simulink model "wheelleg_simulator"  (R2024b)
settings: Solver=VariableStepAuto  StartTime=0.0  StopTime=15.0  RelTol=1e-3
undefined symbols (not defined in the file): eta_l, g, mb, ml, Rl, X, Y, Z
libraries: sm_lib x92, nesl_utility x27, simulink x8, slpidlib x2
(part 1 of 3)
settings Model: Creator=Ame  LastModifiedBy=Ame

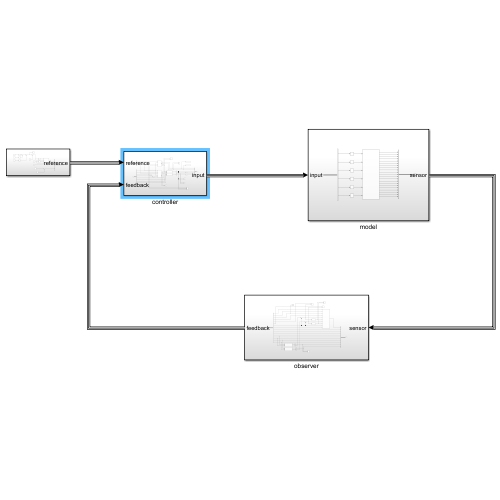
[thumbnail: Simulink's stored preview of the top-level diagram]
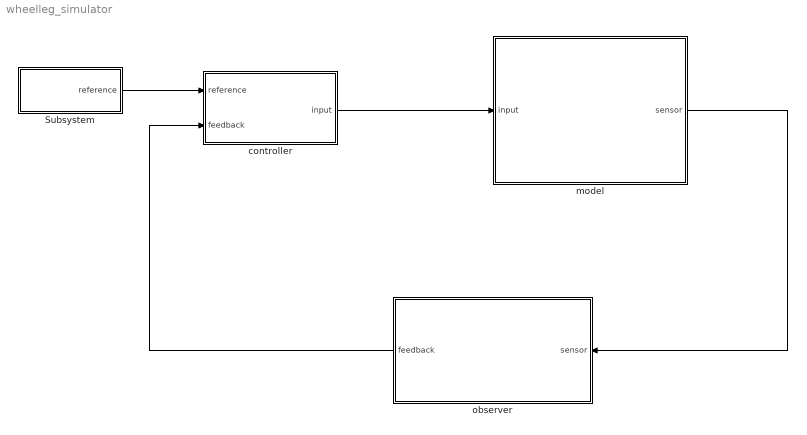
== system wheelleg_simulator ==
  Subsystem : Subsystem
  controller : Subsystem
  model : Subsystem
  observer : Subsystem
  wires:
  model/1(sensor) -> observer/1(sensor)
  observer/1(feedback) -> controller/2(feedback)
  controller/1(input) -> model/1(input)
  Subsystem/1(reference) -> controller/1(reference)

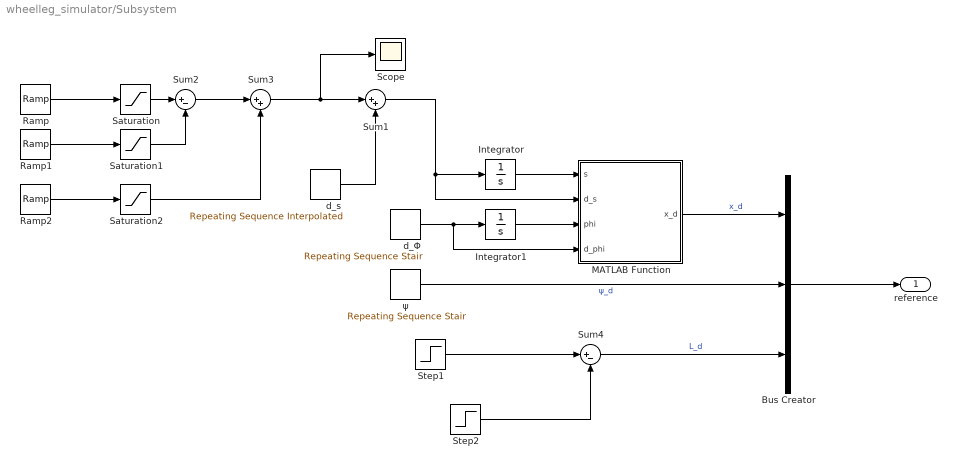
== system wheelleg_simulator/Subsystem ==
  Bus Creator : BusCreator  Inputs=3
  Integrator : Integrator
  Integrator1 : Integrator
  MATLAB Function : MATLAB Function  TreatAsAtomicUnit=on
  Ramp : simulink/Sources/Ramp  slope=0.3  start=0  InitialOutput=0
  Ramp1 : simulink/Sources/Ramp  slope=0.3  start=12  InitialOutput=0
  Ramp2 : simulink/Sources/Ramp  slope=0.3  start=5.5  InitialOutput=0
  Saturation : Saturate  UpperLimit=1.5
  Saturation1 : Saturate  UpperLimit=1  LowerLimit=-0.21
  Saturation2 : Saturate  UpperLimit=0.6
  Scope : Scope
  Step1 : Step  Time=9.0  Before=0.25  After=0.45  SampleTime=0
  Step2 : Step  Time=9.15  After=0.2  SampleTime=0
  Sum1 : Sum  Inputs=|++
  Sum2 : Sum  Inputs=|+-
  Sum3 : Sum  Inputs=|++
  Sum4 : Sum  Inputs=|+-
  d_s : simulink/Sources/Repeating Sequence Interpolated  OutValues=[0 0 0 0 0 0].'  TimeValues=[0 2 3 4 5 6 ].'  LookUpMeth=Interpolation-Use End Values  tsamp=0.01  OutMin=[]  OutMax=[]  OutDataTypeStr=double  OutputDataTypeScalingMode=double  OutDataType=fixdt(0,8)  OutScaling=2^-10
  d_Φ : simulink/Sources/Repeating Sequence Stair  OutValues=[0].'  tsamp=2  OutMin=[]  OutMax=[]  OutDataTypeStr=double  OutputDataTypeScalingMode=double  OutDataType=fixdt(0,8)  ConRadixGroup=Best Precision: Vector-wise  OutScaling=2^-12
  ψ : simulink/Sources/Repeating Sequence Stair  OutValues=[0].'  tsamp=2  OutMin=[]  OutMax=[]  OutDataTypeStr=double  OutputDataTypeScalingMode=double  OutDataType=fixdt(0,8)  ConRadixGroup=Best Precision: Vector-wise  OutScaling=2^-12
  reference : Outport
  wires:
  Bus Creator/1 -> reference/1
  MATLAB Function/1(x_d) -> Bus Creator/1  "x_d"
  ψ/1 -> Bus Creator/2  "ψ_d"
  Integrator/1 -> MATLAB Function/1(s)
  d_Φ/1 -> MATLAB Function/4(d_phi), Integrator1/1
  Integrator1/1 -> MATLAB Function/3(phi)
  Ramp/1 -> Saturation/1
  d_s/1 -> Sum1/2
  Sum1/1 -> MATLAB Function/2(d_s), Integrator/1
  Saturation/1 -> Sum2/1
  Ramp1/1 -> Saturation1/1
  Saturation1/1 -> Sum2/2
  Step1/1 -> Sum4/1
  Sum4/1 -> Bus Creator/3  "L_d"
  Step2/1 -> Sum4/2
  Saturation2/1 -> Sum3/2
  Ramp2/1 -> Saturation2/1
  Sum2/1 -> Sum3/1
  Sum3/1 -> Scope/1, Sum1/1

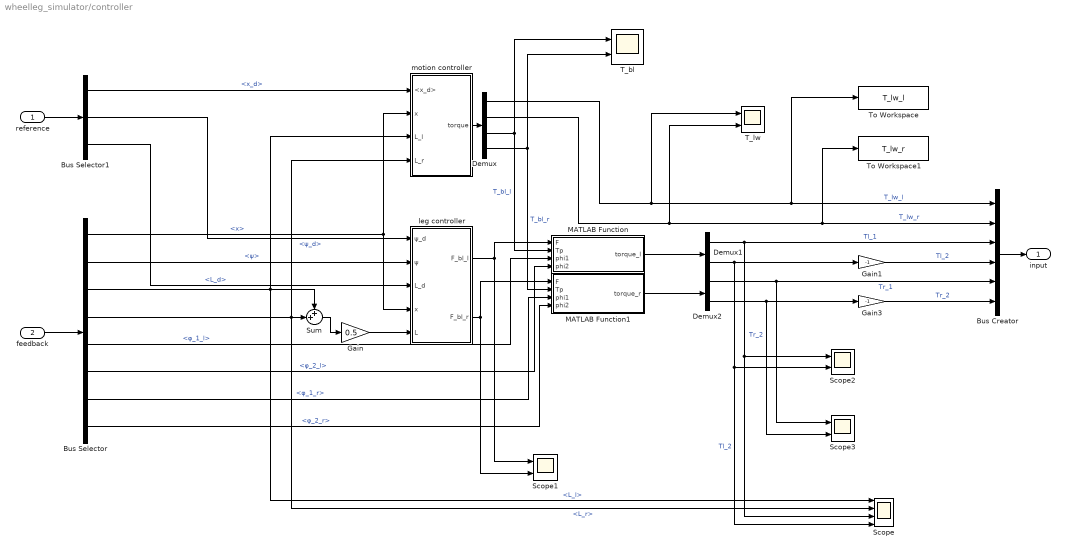
== system wheelleg_simulator/controller ==
  reference : Inport
  feedback : Inport  Port=2
  Bus Creator : BusCreator  Inputs=6
  Bus Selector : BusSelector  OutputSignals=x,ψ,L_l,L_r,φ_1_l,φ_2_l,φ_1_r,φ_2_r
  Bus Selector1 : BusSelector  OutputSignals=x_d,ψ_d,L_d
  Demux : Demux
  Demux1 : Demux  Outputs=2
  Demux2 : Demux  Outputs=2
  Gain : Gain  Gain=0.5
  Gain1 : Gain  Gain=-1
  Gain3 : Gain  Gain=-1
  MATLAB Function : MATLAB Function  TreatAsAtomicUnit=on
  MATLAB Function1 : MATLAB Function  TreatAsAtomicUnit=on
  Scope : Scope  NumInputPorts=4
  Scope1 : Scope  NumInputPorts=2
  Scope2 : Scope  NumInputPorts=2
  Scope3 : Scope  NumInputPorts=2
  Sum : Sum  Inputs=++|
  T_bl : Scope  NumInputPorts=2
  T_lw : Scope  NumInputPorts=2
  To Workspace : ToWorkspace  VariableName=T_lw_l  SaveFormat=Timeseries  SampleTime=-1
  To Workspace1 : ToWorkspace  VariableName=T_lw_r  SaveFormat=Timeseries  SampleTime=-1
  leg controller : Subsystem
  motion controller : Subsystem
  input : Outport
  wires:
  feedback/1 -> Bus Selector/1
  Bus Selector/1 -> motion controller/2(x), leg controller/4(x)  "<x>"
  Bus Selector/2 -> leg controller/2(ψ)  "<ψ>"
  Bus Selector/3 -> Scope/1, motion controller/3(L_l), Sum/1  "<L_l>"
  Bus Selector/4 -> motion controller/4(L_r), Sum/2, Scope/2  "<L_r>"
  reference/1 -> Bus Selector1/1
  Bus Selector1/1 -> motion controller/1(<x_d>)  "<x_d>"
  Bus Selector1/2 -> leg controller/1(ψ_d)  "<ψ_d>"
  Bus Selector1/3 -> leg controller/3(L_d)  "<L_d>"
  motion controller/1(torque) -> Demux/1
  Demux/1 -> To Workspace/1, Bus Creator/1, T_lw/1  "T_lw_l"
  Demux/3 -> MATLAB Function/2(Tp), T_bl/1  "T_bl_l"
  Demux/4 -> MATLAB Function1/2(Tp), T_bl/2  "T_bl_r"
  Bus Selector/5 -> MATLAB Function/3(phi1)  "<φ_1_l>"
  Bus Selector/6 -> MATLAB Function/4(phi2)  "<φ_2_l>"
  Bus Selector/7 -> MATLAB Function1/3(phi1)  "<φ_1_r>"
  Bus Selector/8 -> MATLAB Function1/4(phi2)  "<φ_2_r>"
  Bus Creator/1 -> input/1
  MATLAB Function/1(torque_l) -> Demux1/1
  MATLAB Function1/1(torque_r) -> Demux2/1
  Demux2/2 -> Scope3/2, Gain3/1  "Tr_2"
  Demux1/1 -> Bus Creator/3, Scope2/1, Scope/3  "Tl_1"
  Demux1/2 -> Scope2/2, Scope/4, Gain1/1  "Tl_2"
  Demux2/1 -> Bus Creator/5, Scope3/1  "Tr_1"
  leg controller/1(F_bl_l) -> MATLAB Function/1(F), Scope1/1
  Demux/2 -> To Workspace1/1, Bus Creator/2, T_lw/2  "T_lw_r"
  leg controller/2(F_bl_r) -> MATLAB Function1/1(F), Scope1/2
  Sum/1 -> Gain/1
  Gain1/1 -> Bus Creator/4  "Tl_2"
  Gain3/1 -> Bus Creator/6  "Tr_2"
  Gain/1 -> leg controller/5(L)

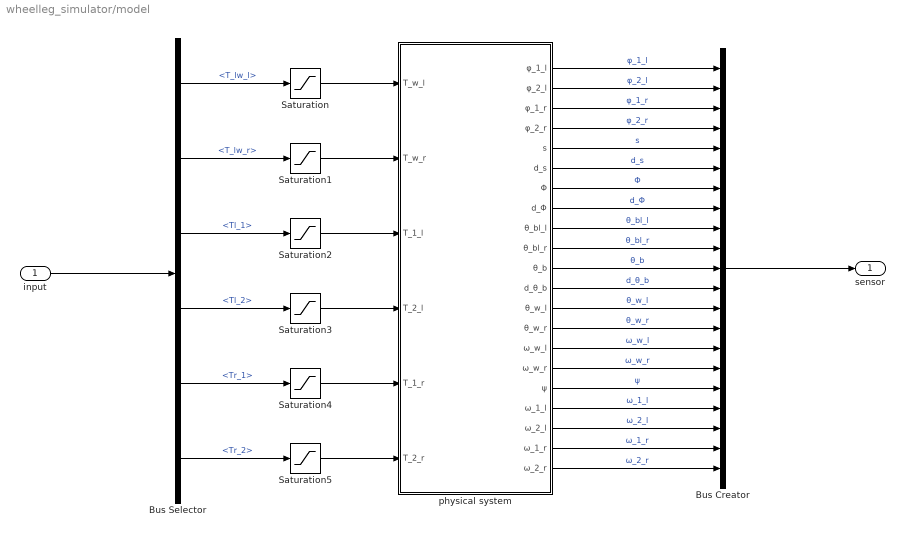
== system wheelleg_simulator/model ==
  input : Inport
  Bus Creator : BusCreator  Inputs=21
  Bus Selector : BusSelector  OutputSignals=T_lw_l,T_lw_r,Tl_1,Tl_2,Tr_1,Tr_2
  Saturation{,1..5} (6 alike) : Saturate  UpperLimit=100  LowerLimit=-100
  physical system : Subsystem
  sensor : Outport
  wires:
  Bus Creator/1 -> sensor/1
  input/1 -> Bus Selector/1
  Bus Selector/1 -> Saturation/1  "<T_lw_l>"
  Bus Selector/2 -> Saturation1/1  "<T_lw_r>"
  physical system/1(φ_1_l) -> Bus Creator/1  "φ_1_l"
  physical system/2(φ_2_l) -> Bus Creator/2  "φ_2_l"
  physical system/3(φ_1_r) -> Bus Creator/3  "φ_1_r"
  physical system/4(φ_2_r) -> Bus Creator/4  "φ_2_r"
  physical system/5(s) -> Bus Creator/5  "s"
  physical system/6(d_s) -> Bus Creator/6  "d_s"
  physical system/7(Φ) -> Bus Creator/7  "Φ"
  physical system/8(d_Φ) -> Bus Creator/8  "d_Φ"
  physical system/9(θ_bl_l) -> Bus Creator/9  "θ_bl_l"
  physical system/10(θ_bl_r) -> Bus Creator/10  "θ_bl_r"
  physical system/11(θ_b) -> Bus Creator/11  "θ_b"
  physical system/12(d_θ_b) -> Bus Creator/12  "d_θ_b"
  physical system/13(θ_w_l) -> Bus Creator/13  "θ_w_l"
  physical system/14(θ_w_r) -> Bus Creator/14  "θ_w_r"
  physical system/15(ω_w_l) -> Bus Creator/15  "ω_w_l"
  physical system/16(ω_w_r) -> Bus Creator/16  "ω_w_r"
  physical system/17(ψ) -> Bus Creator/17  "ψ"
  physical system/18(ω_1_l) -> Bus Creator/18  "ω_1_l"
  physical system/19(ω_2_l) -> Bus Creator/19  "ω_2_l"
  physical system/20(ω_1_r) -> Bus Creator/20  "ω_1_r"
  physical system/21(ω_2_r) -> Bus Creator/21  "ω_2_r"
  Saturation/1 -> physical system/1(T_w_l)
  Saturation2/1 -> physical system/3(T_1_l)
  Saturation1/1 -> physical system/2(T_w_r)
  Saturation3/1 -> physical system/4(T_2_l)
  Saturation4/1 -> physical system/5(T_1_r)
  Saturation5/1 -> physical system/6(T_2_r)
  Bus Selector/3 -> Saturation2/1  "<Tl_1>"
  Bus Selector/4 -> Saturation3/1  "<Tl_2>"
  Bus Selector/5 -> Saturation4/1  "<Tr_1>"
  Bus Selector/6 -> Saturation5/1  "<Tr_2>"

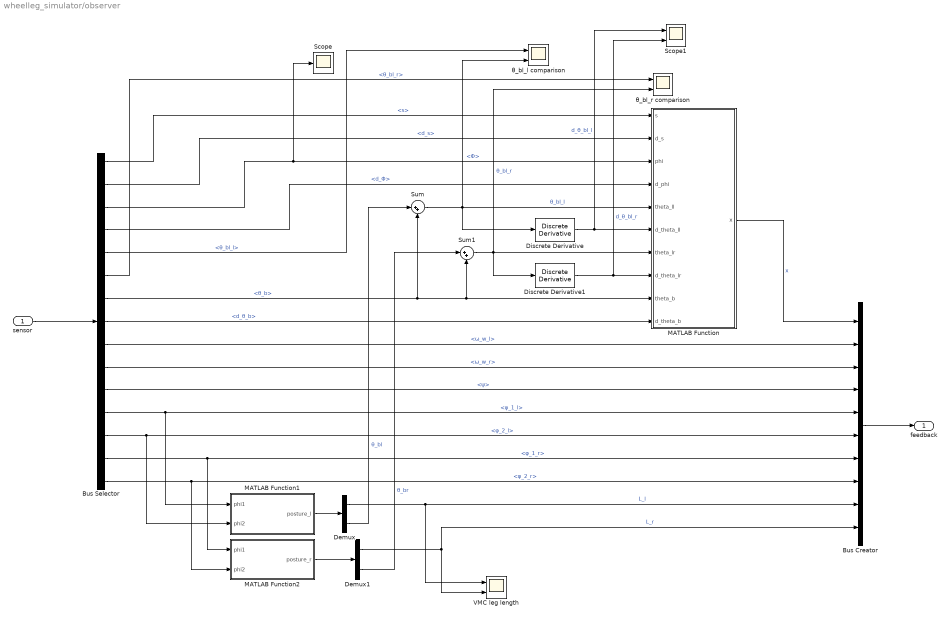
== system wheelleg_simulator/observer ==
  sensor : Inport
  Bus Creator : BusCreator  Inputs=10
  Bus Selector : BusSelector  OutputSignals=s,d_s,Φ,d_Φ,θ_bl_l,θ_bl_r,θ_b,d_θ_b,ω_w_l,ω_w_r,ψ,φ_1_l,φ_2_l,φ_1_r,φ_2_r
  Demux : Demux  Outputs=2
  Demux1 : Demux  Outputs=2
  Discrete Derivative : simulink/Discrete/Discrete Derivative  gainval=1.0  ICPrevScaledInput=0.0  OutMin=[]  OutMax=[]  OutDataType=fixdt(1, 16)  OutScaling=2^-10  DoSatur=off
  Discrete Derivative1 : simulink/Discrete/Discrete Derivative  gainval=1.0  ICPrevScaledInput=0.0  OutMin=[]  OutMax=[]  OutDataType=fixdt(1, 16)  OutScaling=2^-10  DoSatur=off
  MATLAB Function : MATLAB Function  TreatAsAtomicUnit=on
  MATLAB Function1 : MATLAB Function  TreatAsAtomicUnit=on
  MATLAB Function2 : MATLAB Function  TreatAsAtomicUnit=on
  Scope : Scope
  Scope1 : Scope  NumInputPorts=2
  Sum : Sum  Inputs=|++
  Sum1 : Sum  Inputs=|++
  VMC leg length : Scope  NumInputPorts=2
  θ_bl_l comparison : Scope  NumInputPorts=2
  θ_bl_r comparison : Scope  NumInputPorts=2
  feedback : Outport
  wires:
  sensor/1 -> Bus Selector/1
  Bus Creator/1 -> feedback/1
  Sum/1 -> MATLAB Function/5(theta_ll), Discrete Derivative/1, θ_bl_l comparison/2  "θ_bl_l"
  Bus Selector/1 -> MATLAB Function/1(s)  "<s>"
  Bus Selector/2 -> MATLAB Function/2(d_s)  "<d_s>"
  Bus Selector/3 -> Scope/1, MATLAB Function/3(phi)  "<Φ>"
  Bus Selector/4 -> MATLAB Function/4(d_phi)  "<d_Φ>"
  Bus Selector/7 -> MATLAB Function/9(theta_b), Sum1/2, Sum/2  "<θ_b>"
  Bus Selector/8 -> MATLAB Function/10(d_theta_b)  "<d_θ_b>"
  Sum1/1 -> MATLAB Function/7(theta_lr), Discrete Derivative1/1, θ_bl_r comparison/2  "θ_bl_r"
  Bus Selector/9 -> Bus Creator/2  "<ω_w_l>"
  Bus Selector/10 -> Bus Creator/3  "<ω_w_r>"
  Bus Selector/11 -> Bus Creator/4  "<ψ>"
  Bus Selector/12 -> MATLAB Function1/1(phi1), Bus Creator/5  "<φ_1_l>"
  Bus Selector/13 -> MATLAB Function1/2(phi2), Bus Creator/6  "<φ_2_l>"
  Bus Selector/14 -> MATLAB Function2/1(phi1), Bus Creator/7  "<φ_1_r>"
  Bus Selector/15 -> MATLAB Function2/2(phi2), Bus Creator/8  "<φ_2_r>"
  MATLAB Function/1(x) -> Bus Creator/1  "x"
  Discrete Derivative/1 -> MATLAB Function/6(d_theta_ll), Scope1/1  "d_θ_bl_l"
  Discrete Derivative1/1 -> Scope1/2, MATLAB Function/8(d_theta_lr)  "d_θ_bl_r"
  MATLAB Function1/1(posture_l) -> Demux/1
  Demux/1 -> VMC leg length/1, Bus Creator/9  "L_l"
  Demux/2 -> Sum/1  "θ_bl"
  MATLAB Function2/1(posture_r) -> Demux1/1
  Demux1/1 -> Bus Creator/10, VMC leg length/2  "L_r"
  Demux1/2 -> Sum1/1  "θ_br"
  Bus Selector/5 -> θ_bl_l comparison/1  "<θ_bl_l>"
  Bus Selector/6 -> θ_bl_r comparison/1  "<θ_bl_r>"

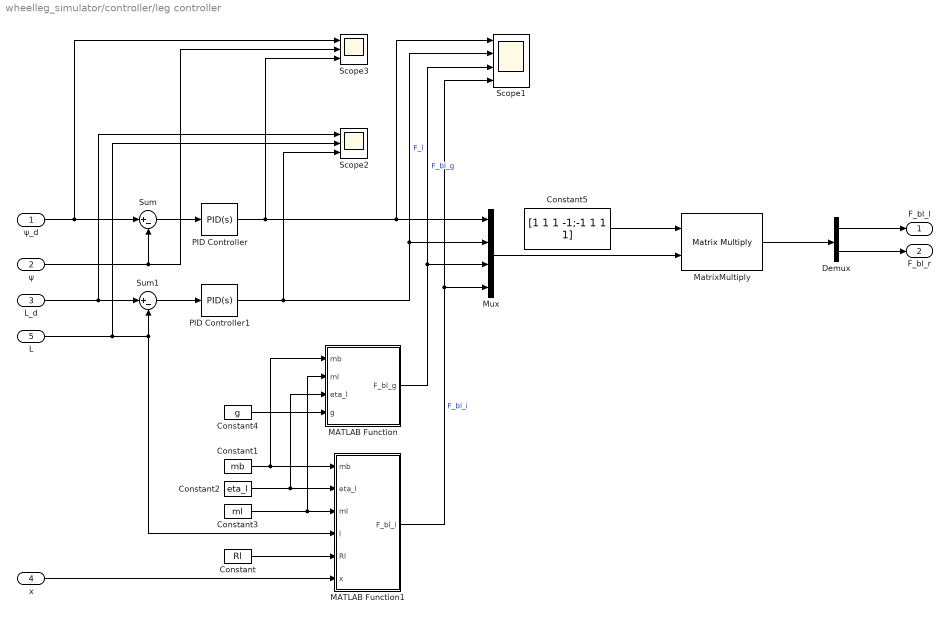
== system wheelleg_simulator/controller/leg controller ==
  ψ_d : Inport
  ψ : Inport  Port=2
  L_d : Inport  Port=3
  x : Inport  Port=4
  L : Inport  Port=5
  Constant : Constant  Value=Rl
  Constant1 : Constant  Value=mb
  Constant2 : Constant  Value=eta_l
  Constant3 : Constant  Value=ml
  Constant4 : Constant  Value=g
  Constant5 : Constant  Value=[1 1 1 -1;-1 1 1 1]
  Demux : Demux  Outputs=2
  MATLAB Function : MATLAB Function  TreatAsAtomicUnit=on
  MATLAB Function1 : MATLAB Function  TreatAsAtomicUnit=on
  MatrixMultiply : Product  Multiplication=Matrix(*)
  Mux : Mux
  PID Controller : slpidlib/PID Controller  Controller=PID  Form=Parallel  TimeDomain=Continuous-time  UseExternalTs=off  SampleTime=-1  IntegratorMethod=Forward Euler  FilterMethod=Forward Euler  ControllerParametersSource=internal  P=300  I=0.0003  UseKiTs=off  D=10  UseExternalDerivativeSource=off  N=100  UseFilter=on  TunerSelectOption=Transfer Function Based (PID Tuner App)  InitialConditionSource=internal  InitialConditionForIntegrator=0  InitialConditionForFilter=0  DifferentiatorICPrevScaledInput=0  ExternalReset=none  TrackingMode=off  Kt=1  LimitOutput=off  SatLimitsSource=internal  UpperSaturationLimit=inf  LowerSaturationLimit=-inf  LinearizeAsGain=on  AntiWindupMode=none  Kb=1  LimitIntegrator=off  UpperIntegratorSaturationLimit=inf  LowerIntegratorSaturationLimit=-inf  POutMin=[]  POutMax=[]  IOutMin=[]  IOutMax=[]  DOutMin=[]  DOutMax=[]  NOutMin=[]  NOutMax=[]  SumOutMin=[]  SumOutMax=[]  SaturationOutMin=[]  SaturationOutMax=[]  PParamMin=[]  PParamMax=[]  IParamMin=[]  IParamMax=[]  DParamMin=[]  DParamMax=[]  NParamMin=[]  NParamMax=[]  KbParamMin=[]  KbParamMax=[]  KtParamMin=[]  KtParamMax=[]  KbOutMin=[]  KbOutMax=[]  KtOutMin=[]  KtOutMax=[]  IntegratorOutMin=[]  IntegratorOutMax=[]  FilterOutMin=[]  FilterOutMax=[]  SumI1OutMin=[]  SumI1OutMax=[]  SumI2OutMin=[]  SumI2OutMax=[]  SumI3OutMin=[]  SumI3OutMax=[]  SumI4OutMin=[]  SumI4OutMax=[]  SumDOutMin=[]  SumDOutMax=[]  DifferentiatorOutMin=[]  DifferentiatorOutMax=[]  FilterDiffOutCoefMin=[]  FilterDiffOutCoefMax=[]  ReciprocalOutMin=[]  ReciprocalOutMax=[]  SumDenOutMin=[]  SumDenOutMax=[]  SumNumOutMin=[]  SumNumOutMax=[]  DivideOutMin=[]  DivideOutMax=[]  UdiffTsProdOutMin=[]  UdiffTsProdOutMax=[]  NTsProdOutMin=[]  NTsProdOutMax=[]  UintegralTsProdOutMin=[]  UintegralTsProdOutMax=[]  UngainTsProdOutMin=[]  UngainTsProdOutMax=[]  ClampingZeroOutDataTypeStr=Inherit: Inherit via back propagation  ClampingZeroOutMin=[]  ClampingZeroOutMax=[]  FilterDenConstantOutDataTypeStr=Inherit: Inherit via back propagation  FilterDenConstantOutMin=[]  FilterDenConstantOutMax=[]  PCopyOutDataTypeStr=Inherit: Inherit via back propagation  PCopyOutMin=[]  PCopyOutMax=[]  NCopyOutDataTypeStr=Inherit: Inherit via back propagation  NCopyOutMin=[]  NCopyOutMax=[]  IntegratorContinuousStateAttributes=''  IntegratorStateMustResolveToSignalObject=off  IntegratorRTWStateStorageClass=Auto  FilterContinuousStateAttributes=''  FilterStateMustResolveToSignalObject=off  FilterRTWStateStorageClass=Auto  ParallelPVariant=InternalParameters  IdealPVariant=Disabled  IVariant=InternalParameters  DVariant=InternalParameters  IntegratorVariant=Continuous  SatVariant=Disabled  AWVariant=Passthrough  PCopyVariant=Disabled  TRVariant=Disabled  FdbkBlocksVariant=Forward  IdealPFdbkVariant=Disabled  SatFdbkVariant=Disabled  DerivativeFilterVariant=ContFilter  NVariant=InternalParameters  NCopyVariant=Disabled  FilterICVariant=InternalICsFilter  IntegratorICVariant=InternalICs  ExternalResetVariant=Disabled  TRSumVariant=Passthrough  SumFdbkVariant=Disabled  SumVariant=Sum_PID  TsampFilterVariant=InternalTs  TsampNgainVariant=Passthrough  TsampIntegralVariant=Disabled_SignalSpec  ExternalSaturationOutDataTypeStr=Inherit: Same as second input  DerivativeSourceVariant=ErrorSignal  PreIntVariant=InternalPreInt
  PID Controller1 : slpidlib/PID Controller  Controller=PID  Form=Parallel  TimeDomain=Continuous-time  UseExternalTs=off  SampleTime=-1  IntegratorMethod=Forward Euler  FilterMethod=Forward Euler  ControllerParametersSource=internal  P=2000  I=4  UseKiTs=off  D=20  UseExternalDerivativeSource=off  N=100  UseFilter=on  TunerSelectOption=Transfer Function Based (PID Tuner App)  InitialConditionSource=internal  InitialConditionForIntegrator=0  InitialConditionForFilter=0  DifferentiatorICPrevScaledInput=0  ExternalReset=none  TrackingMode=off  Kt=1  LimitOutput=off  SatLimitsSource=internal  UpperSaturationLimit=inf  LowerSaturationLimit=-inf  LinearizeAsGain=on  AntiWindupMode=none  Kb=1  LimitIntegrator=off  UpperIntegratorSaturationLimit=inf  LowerIntegratorSaturationLimit=-inf  POutMin=[]  POutMax=[]  IOutMin=[]  IOutMax=[]  DOutMin=[]  DOutMax=[]  NOutMin=[]  NOutMax=[]  SumOutMin=[]  SumOutMax=[]  SaturationOutMin=[]  SaturationOutMax=[]  PParamMin=[]  PParamMax=[]  IParamMin=[]  IParamMax=[]  DParamMin=[]  DParamMax=[]  NParamMin=[]  NParamMax=[]  KbParamMin=[]  KbParamMax=[]  KtParamMin=[]  KtParamMax=[]  KbOutMin=[]  KbOutMax=[]  KtOutMin=[]  KtOutMax=[]  IntegratorOutMin=[]  IntegratorOutMax=[]  FilterOutMin=[]  FilterOutMax=[]  SumI1OutMin=[]  SumI1OutMax=[]  SumI2OutMin=[]  SumI2OutMax=[]  SumI3OutMin=[]  SumI3OutMax=[]  SumI4OutMin=[]  SumI4OutMax=[]  SumDOutMin=[]  SumDOutMax=[]  DifferentiatorOutMin=[]  DifferentiatorOutMax=[]  FilterDiffOutCoefMin=[]  FilterDiffOutCoefMax=[]  ReciprocalOutMin=[]  ReciprocalOutMax=[]  SumDenOutMin=[]  SumDenOutMax=[]  SumNumOutMin=[]  SumNumOutMax=[]  DivideOutMin=[]  DivideOutMax=[]  UdiffTsProdOutMin=[]  UdiffTsProdOutMax=[]  NTsProdOutMin=[]  NTsProdOutMax=[]  UintegralTsProdOutMin=[]  UintegralTsProdOutMax=[]  UngainTsProdOutMin=[]  UngainTsProdOutMax=[]  ClampingZeroOutDataTypeStr=Inherit: Inherit via back propagation  ClampingZeroOutMin=[]  ClampingZeroOutMax=[]  FilterDenConstantOutDataTypeStr=Inherit: Inherit via back propagation  FilterDenConstantOutMin=[]  FilterDenConstantOutMax=[]  PCopyOutDataTypeStr=Inherit: Inherit via back propagation  PCopyOutMin=[]  PCopyOutMax=[]  NCopyOutDataTypeStr=Inherit: Inherit via back propagation  NCopyOutMin=[]  NCopyOutMax=[]  IntegratorContinuousStateAttributes=''  IntegratorStateMustResolveToSignalObject=off  IntegratorRTWStateStorageClass=Auto  FilterContinuousStateAttributes=''  FilterStateMustResolveToSignalObject=off  FilterRTWStateStorageClass=Auto  ParallelPVariant=InternalParameters  IdealPVariant=Disabled  IVariant=InternalParameters  DVariant=InternalParameters  IntegratorVariant=Continuous  SatVariant=Disabled  AWVariant=Passthrough  PCopyVariant=Disabled  TRVariant=Disabled  FdbkBlocksVariant=Forward  IdealPFdbkVariant=Disabled  SatFdbkVariant=Disabled  DerivativeFilterVariant=ContFilter  NVariant=InternalParameters  NCopyVariant=Disabled  FilterICVariant=InternalICsFilter  IntegratorICVariant=InternalICs  ExternalResetVariant=Disabled  TRSumVariant=Passthrough  SumFdbkVariant=Disabled  SumVariant=Sum_PID  TsampFilterVariant=InternalTs  TsampNgainVariant=Passthrough  TsampIntegralVariant=Disabled_SignalSpec  ExternalSaturationOutDataTypeStr=Inherit: Same as second input  DerivativeSourceVariant=ErrorSignal  PreIntVariant=InternalPreInt
  Scope1 : Scope  NumInputPorts=4
  Scope2 : Scope  NumInputPorts=3
  Scope3 : Scope  NumInputPorts=3
  Sum : Sum  Inputs=|+-
  Sum1 : Sum  Inputs=|+-
  F_bl_l : Outport
  F_bl_r : Outport  Port=2
  wires:
  ψ_d/1 -> Scope3/1, Sum/1
  L_d/1 -> Scope2/1, Sum1/1
  ψ/1 -> Scope3/2, Sum/2
  L/1 -> Scope2/2, MATLAB Function1/4(l), Sum1/2
  MatrixMultiply/1 -> Demux/1
  Demux/1 -> F_bl_l/1
  Demux/2 -> F_bl_r/1
  Sum/1 -> PID Controller/1
  Sum1/1 -> PID Controller1/1
  PID Controller/1 -> Scope1/1, Mux/1, Scope3/3
  PID Controller1/1 -> Scope2/3, Scope1/2, Mux/2  "F_l"
  Constant1/1 -> MATLAB Function/1(mb), MATLAB Function1/1(mb)
  Constant2/1 -> MATLAB Function/3(eta_l), MATLAB Function1/2(eta_l)
  Constant3/1 -> MATLAB Function/2(ml), MATLAB Function1/3(ml)
  Constant4/1 -> MATLAB Function/4(g)
  Constant/1 -> MATLAB Function1/5(Rl)
  MATLAB Function1/1(F_bl_i) -> Scope1/4, Mux/4  "F_bl_i"
  MATLAB Function/1(F_bl_g) -> Scope1/3, Mux/3  "F_bl_g"
  Mux/1 -> MatrixMultiply/2
  Constant5/1 -> MatrixMultiply/1
  x/1 -> MATLAB Function1/6(x)

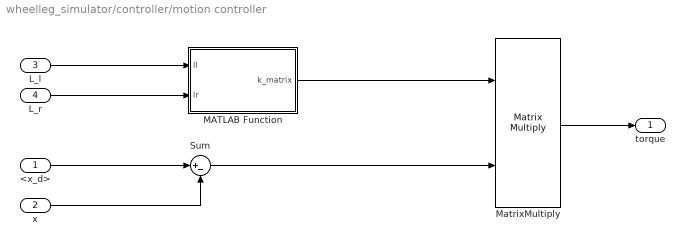
== system wheelleg_simulator/controller/motion controller ==
  <x_d> : Inport
  x : Inport  Port=2
  L_l : Inport  Port=3
  L_r : Inport  Port=4
  MATLAB Function : MATLAB Function  TreatAsAtomicUnit=on
  MatrixMultiply : Product  Multiplication=Matrix(*)
  Sum : Sum  Inputs=|+-
  torque : Outport
  wires:
  L_l/1 -> MATLAB Function/1(ll)
  L_r/1 -> MATLAB Function/2(lr)
  MATLAB Function/1(k_matrix) -> MatrixMultiply/1
  MatrixMultiply/1 -> torque/1
  x/1 -> Sum/2
  <x_d>/1 -> Sum/1
  Sum/1 -> MatrixMultiply/2

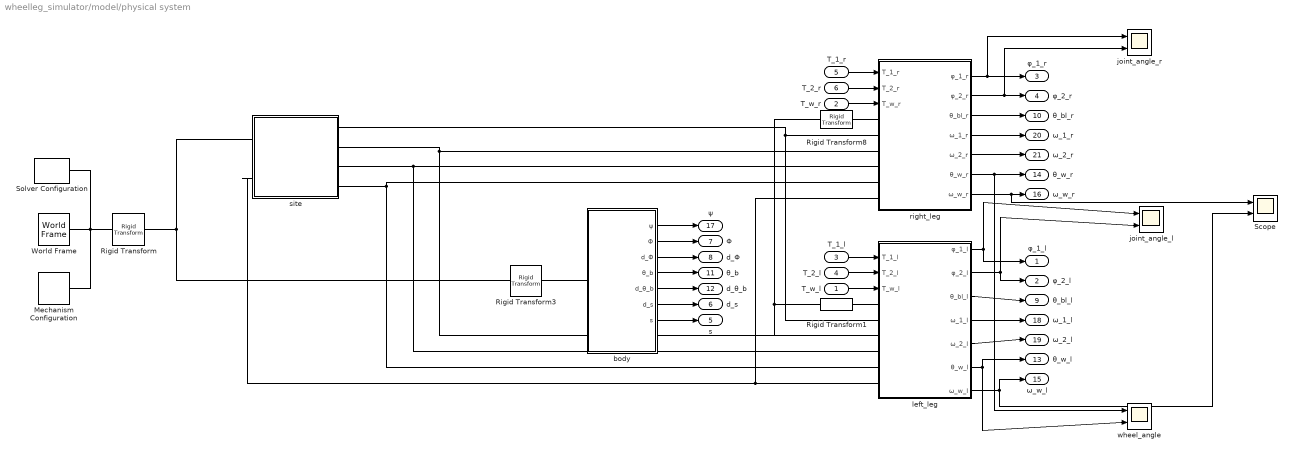
== system wheelleg_simulator/model/physical system ==
  T_w_l : Inport
  T_w_r : Inport  Port=2
  T_1_l : Inport  Port=3
  T_2_l : Inport  Port=4
  T_1_r : Inport  Port=5
  T_2_r : Inport  Port=6
  Mechanism Configuration : sm_lib/Utilities/Mechanism Configuration  UniformGravity=Constant  GravityVector=[0 0 -9.80665]  GravityVectorUnits=m/s^2  LinearizationDelta=0.001  JointModeTransitionNonlinearIterations=2
  Rigid Transform : sm_lib/Frames and Transforms/Rigid Transform  RotationMethod=StandardAxis  FollAlignAxisA=+X  BaseAlignAxisA=+Y  FollAlignAxisB=+Y  BaseAlignAxisB=+Z  RotationStandardAxis=-X  RotationAngle=90  RotationAngleUnits=deg  RotationArbitraryAxis=[0 0 1]  RotationSequenceAxes=FollowerAxes  RotationSequence=XYX  RotationSequenceAngles=[0 0 0]  RotationSequenceAnglesUnits=deg  RotationMatrix=[1 0 0;0 0 1;0 1 0]  Quaternion=[1 0 0 0]  TranslationMethod=None  TranslationCartesianOffset=[0 0 0]  TranslationCartesianOffsetUnits=m  TranslationStandardAxis=+Z  TranslationStandardOffset=0  TranslationStandardOffsetUnits=m  TranslationROffset=0  TranslationROffsetUnits=m  TranslationThetaOffset=0  TranslationThetaOffsetUnits=deg  TranslationZOffset=0  TranslationZOffsetUnits=m
  Rigid Transform1 : sm_lib/Frames and Transforms/Rigid Transform  RotationMethod=None  FollAlignAxisA=+X  BaseAlignAxisA=+Y  FollAlignAxisB=+Y  BaseAlignAxisB=+Z  RotationStandardAxis=+Z  RotationAngle=0  RotationAngleUnits=deg  RotationArbitraryAxis=[0 0 1]  RotationSequenceAxes=FollowerAxes  RotationSequence=XYX  RotationSequenceAngles=[0 0 0]  RotationSequenceAnglesUnits=deg  RotationMatrix=[1 0 0;0 1 0;0 0 1]  Quaternion=[1 0 0 0]  TranslationMethod=StandardAxis  TranslationCartesianOffset=[0 0 0]  TranslationCartesianOffsetUnits=m  TranslationStandardAxis=+Z  TranslationStandardOffset=0.2  TranslationStandardOffsetUnits=m  TranslationROffset=0  TranslationROffsetUnits=m  TranslationThetaOffset=0  TranslationThetaOffsetUnits=deg  TranslationZOffset=0  TranslationZOffsetUnits=m
  Rigid Transform3 : sm_lib/Frames and Transforms/Rigid Transform  RotationMethod=None  FollAlignAxisA=+X  BaseAlignAxisA=+Y  FollAlignAxisB=+Y  BaseAlignAxisB=+Z  RotationStandardAxis=+Y  RotationAngle=30  RotationAngleUnits=deg  RotationArbitraryAxis=[0 0 1]  RotationSequenceAxes=FollowerAxes  RotationSequence=XYX  RotationSequenceAngles=[0 0 0]  RotationSequenceAnglesUnits=deg  RotationMatrix=[1 0 0;0 0 1;0 1 0]  Quaternion=[1 0 0 0]  TranslationMethod=StandardAxis  TranslationCartesianOffset=[0 0 0]  TranslationCartesianOffsetUnits=m  TranslationStandardAxis=-Y  TranslationStandardOffset=0.5  TranslationStandardOffsetUnits=m  TranslationROffset=0  TranslationROffsetUnits=m  TranslationThetaOffset=0  TranslationThetaOffsetUnits=deg  TranslationZOffset=0  TranslationZOffsetUnits=m
  Rigid Transform8 : sm_lib/Frames and Transforms/Rigid Transform  RotationMethod=None  FollAlignAxisA=+X  BaseAlignAxisA=+Y  FollAlignAxisB=+Y  BaseAlignAxisB=+Z  RotationStandardAxis=+Z  RotationAngle=0  RotationAngleUnits=deg  RotationArbitraryAxis=[0 0 1]  RotationSequenceAxes=FollowerAxes  RotationSequence=XYX  RotationSequenceAngles=[0 0 0]  RotationSequenceAnglesUnits=deg  RotationMatrix=[1 0 0;0 1 0;0 0 1]  Quaternion=[1 0 0 0]  TranslationMethod=StandardAxis  TranslationCartesianOffset=[0 0 0]  TranslationCartesianOffsetUnits=m  TranslationStandardAxis=-Z  TranslationStandardOffset=0.2  TranslationStandardOffsetUnits=m  TranslationROffset=0  TranslationROffsetUnits=m  TranslationThetaOffset=0  TranslationThetaOffsetUnits=deg  TranslationZOffset=0  TranslationZOffsetUnits=m
  Scope : Scope  NumInputPorts=2
  Solver Configuration : nesl_utility/Solver Configuration  PhysicalDomain=network_engine_domain  SubClassName=solver  LeftPortType=input  RightPortType=generic  Tones=[]  Harmonics=[]  SimulateNoise=off  Profile=off  UseLocalSampling=off  EnableSwitchedLinearOptims=on  FrequencyDomain=off  UseCCode=off  RelTol=0.001  AbsTol=0.001  MinStep=1e-09  ToWorkspace=off  RevertToSquareIcSolve=off  NumHomotopyIterations=100  PhasorMode=off  PhasorModeNumHarmonics=1  ConsistencySolver=NEWTON_XTOL_AFTER_FTOL  IndexReductionMethod=DerivativeReplacement  DoDC=off  ResidualTolerance=1e-09  ConsistencyTolSource=GLOBAL  ConsistencyAbsTol=0.001  ConsistencyRelTol=0.001  ConsistencyTolFactor=0.001  UseLocalSolver=off  LocalSolverChoice=NE_BACKWARD_EULER_ADVANCER  ResolveIndetEquations=on  FunctionEvalNumThread=1  LocalSolverSampleTime=0.001  DoFixedCost=off  MaxNonlinIter=3  MaxModeIter=2  ComputeImpulses=off  ImpulseIterations=2  LinearAlgebra=auto  LinearAlgebraNumThread=0  EquationFormulation=NE_TIME_EF  DelaysMemoryBudget=1024  AutomaticFiltering=on  FilteringTimeConstant=0.001  PartitionStorageMethod=AS_NEEDED  PartitionMemoryBudget=1024  PartitionMethod=ROBUST  MultibodyUseLocalSolver=off  MultibodyLocalSolverChoice=ODE1  MultibodyLocalSolverSampleTime=0.001
  World Frame : sm_lib/Frames and Transforms/World Frame
  body : Subsystem
  joint_angle_l : Scope  NumInputPorts=2
  joint_angle_r : Scope  NumInputPorts=2
  left_leg : Subsystem
  right_leg : Subsystem
  site : Subsystem
  wheel_angle : Scope  NumInputPorts=2
  φ_1_l : Outport
  φ_2_l : Outport  Port=2
  φ_1_r : Outport  Port=3
  φ_2_r : Outport  Port=4
  s : Outport  Port=5
  d_s : Outport  Port=6
  Φ : Outport  Port=7
  d_Φ : Outport  Port=8
  θ_bl_l : Outport  Port=9
  θ_bl_r : Outport  Port=10
  θ_b : Outport  Port=11
  d_θ_b : Outport  Port=12
  θ_w_l : Outport  Port=13
  θ_w_r : Outport  Port=14
  ω_w_l : Outport  Port=15
  ω_w_r : Outport  Port=16
  ψ : Outport  Port=17
  ω_1_l : Outport  Port=18
  ω_2_l : Outport  Port=19
  ω_1_r : Outport  Port=20
  ω_2_r : Outport  Port=21
  wires:
  left_leg/4(ω_1_l) -> ω_1_l/1
  left_leg/3(θ_bl_l) -> θ_bl_l/1
  left_leg/5(ω_2_l) -> ω_2_l/1
  left_leg/7(ω_w_l) -> ω_w_l/1, Scope/2
  left_leg/6(θ_w_l) -> θ_w_l/1, wheel_angle/2
  right_leg/1(φ_1_r) -> joint_angle_r/1, φ_1_r/1
  right_leg/2(φ_2_r) -> joint_angle_r/2, φ_2_r/1
  right_leg/6(θ_w_r) -> θ_w_r/1, wheel_angle/1
  right_leg/5(ω_2_r) -> ω_2_r/1
  right_leg/7(ω_w_r) -> ω_w_r/1, Scope/1
  right_leg/4(ω_1_r) -> ω_1_r/1
  right_leg/3(θ_bl_r) -> θ_bl_r/1
  body/1(ψ) -> ψ/1
  body/2(Φ) -> Φ/1
  body/3(d_Φ) -> d_Φ/1
  body/4(θ_b) -> θ_b/1
  body/5(d_θ_b) -> d_θ_b/1
  body/6(d_s) -> d_s/1
  body/7(s) -> s/1
  left_leg/1(φ_1_l) -> joint_angle_l/1, φ_1_l/1
  left_leg/2(φ_2_l) -> joint_angle_l/2, φ_2_l/1
  T_w_r/1 -> right_leg/3(T_w_r)
  T_w_l/1 -> left_leg/3(T_w_l)
  T_2_r/1 -> right_leg/2(T_2_r)
  T_1_r/1 -> right_leg/1(T_1_r)
  T_1_l/1 -> left_leg/1(T_1_l)
  T_2_l/1 -> left_leg/2(T_2_l)
  connections:
  World Frame/RConn1 -- Rigid Transform/LConn1 -- Solver Configuration/RConn1 -- Mechanism Configuration/RConn1
  left_leg/LConn1 -- Rigid Transform1/RConn1
  Rigid Transform8/RConn1 -- right_leg/LConn1
  Rigid Transform3/RConn1 -- body/LConn1
  Rigid Transform/RConn1 -- site/LConn1 -- Rigid Transform3/LConn1
  Rigid Transform1/LConn1 -- body/RConn1 -- Rigid Transform8/LConn1
  right_leg/LConn2 -- left_leg/LConn2 -- site/RConn1
  site/RConn2 -- right_leg/LConn3 -- left_leg/LConn3
  site/RConn3 -- right_leg/LConn4 -- left_leg/LConn4
  site/RConn4 -- left_leg/LConn5 -- right_leg/LConn5
  site/LConn2 -- right_leg/LConn6 -- left_leg/LConn6

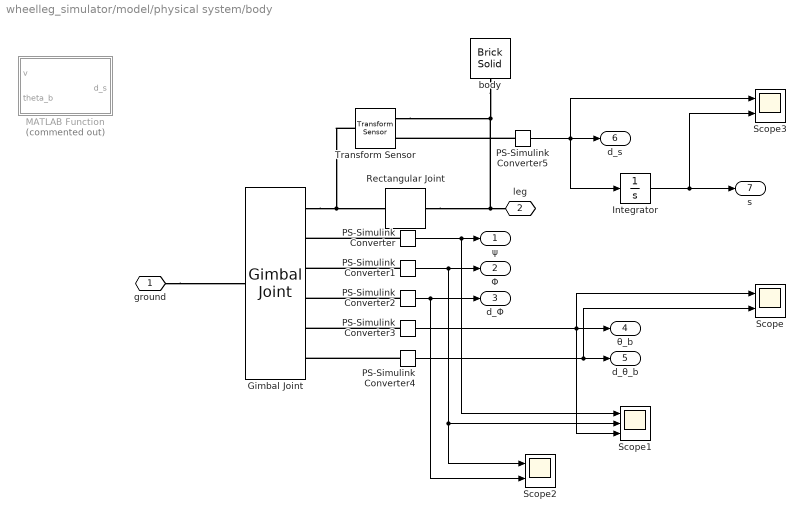
== system wheelleg_simulator/model/physical system/body ==
  Gimbal Joint : sm_lib/Joints/Gimbal Joint  JointMode=Normal  CompositeWrenchDir=FollowerOnBase  CompositeWrenchFrame=BaseFrame  SenseConstraintForce=off  SenseConstraintTorque=off  SenseTotalForce=off  SenseTotalTorque=off  RxPositionTargetSpecify=off  RxPositionTargetPriority=High  RxPositionTargetValue=10  RxPositionTargetValueUnits=deg  RxVelocityTargetSpecify=off  RxVelocityTargetPriority=High  RxVelocityTargetValue=0  RxVelocityTargetValueUnits=deg/s  RxEquilibriumPosition=0  RxEquilibriumPositionUnits=deg  RxSpringStiffness=0  RxSpringStiffnessUnits=N*m/deg  RxDampingCoefficient=0  RxDampingCoefficientUnits=N*m/(deg/s)  RxLowerLimitSpecify=off  RxLowerLimitBound=-90  RxLowerLimitBoundUnits=deg  RxLowerLimitStiffness=1e4  RxLowerLimitStiffnessUnits=N*m/deg  RxLowerLimitDamping=10  RxLowerLimitDampingUnits=N*m/(deg/s)  RxLowerLimitTransitionRegionWidth=0.1  RxLowerLimitTransitionRegionWidthUnits=deg  RxUpperLimitSpecify=off  RxUpperLimitBound=90  RxUpperLimitBoundUnits=deg  RxUpperLimitStiffness=1e4  RxUpperLimitStiffnessUnits=N*m/deg  RxUpperLimitDamping=10  RxUpperLimitDampingUnits=N*m/(deg/s)  RxUpperLimitTransitionRegionWidth=0.1  RxUpperLimitTransitionRegionWidthUnits=deg  RxTorqueActuationMode=NoTorque  RxMotionActuationMode=ComputedMotion  RxSensePosition=on  RxSenseVelocity=off  RxSenseAcceleration=off  RxSenseTorqueForce=off  RxSenseLowerLimitTorqueForce=off  RxSenseUpperLimitTorqueForce=off  RyPositionTargetSpecify=off  RyPositionTargetPriority=High  RyPositionTargetValue=45  RyPositionTargetValueUnits=deg  RyVelocityTargetSpecify=off  RyVelocityTargetPriority=High  RyVelocityTargetValue=0  RyVelocityTargetValueUnits=deg/s  RyEquilibriumPosition=0  RyEquilibriumPositionUnits=deg  RySpringStiffness=0  RySpringStiffnessUnits=N*m/deg  RyDampingCoefficient=0  RyDampingCoefficientUnits=N*m/(deg/s)  RyLowerLimitSpecify=off  RyLowerLimitBound=-90  RyLowerLimitBoundUnits=deg  RyLowerLimitStiffness=1e4  RyLowerLimitStiffnessUnits=N*m/deg  RyLowerLimitDamping=10  RyLowerLimitDampingUnits=N*m/(deg/s)  RyLowerLimitTransitionRegionWidth=0.1  RyLowerLimitTransitionRegionWidthUnits=deg  RyUpperLimitSpecify=off  RyUpperLimitBound=90  RyUpperLimitBoundUnits=deg  RyUpperLimitStiffness=1e4  RyUpperLimitStiffnessUnits=N*m/deg  RyUpperLimitDamping=10  RyUpperLimitDampingUnits=N*m/(deg/s)  RyUpperLimitTransitionRegionWidth=0.1  RyUpperLimitTransitionRegionWidthUnits=deg  RyTorqueActuationMode=NoTorque  RyMotionActuationMode=ComputedMotion  RySensePosition=on  RySenseVelocity=on  RySenseAcceleration=off  RySenseTorqueForce=off  RySenseLowerLimitTorqueForce=off  RySenseUpperLimitTorqueForce=off  RzPositionTargetSpecify=on  RzPositionTargetPriority=High  RzPositionTargetValue=-20  RzPositionTargetValueUnits=deg  RzVelocityTargetSpecify=off  RzVelocityTargetPriority=High  RzVelocityTargetValue=0  RzVelocityTargetValueUnits=deg/s  RzEquilibriumPosition=0  RzEquilibriumPositionUnits=deg  RzSpringStiffness=0  RzSpringStiffnessUnits=N*m/deg  RzDampingCoefficient=0  RzDampingCoefficientUnits=N*m/(deg/s)  RzLowerLimitSpecify=off  RzLowerLimitBound=-90  RzLowerLimitBoundUnits=deg  RzLowerLimitStiffness=1e4  RzLowerLimitStiffnessUnits=N*m/deg  RzLowerLimitDamping=10  RzLowerLimitDampingUnits=N*m/(deg/s)  RzLowerLimitTransitionRegionWidth=0.1  RzLowerLimitTransitionRegionWidthUnits=deg  RzUpperLimitSpecify=off  RzUpperLimitBound=90  RzUpperLimitBoundUnits=deg  RzUpperLimitStiffness=1e4  RzUpperLimitStiffnessUnits=N*m/deg  RzUpperLimitDamping=10  RzUpperLimitDampingUnits=N*m/(deg/s)  RzUpperLimitTransitionRegionWidth=0.1  RzUpperLimitTransitionRegionWidthUnits=deg  RzTorqueActuationMode=NoTorque  RzMotionActuationMode=ComputedMotion  RzSensePosition=on  RzSenseVelocity=on  RzSenseAcceleration=off  RzSenseTorqueForce=off  RzSenseLowerLimitTorqueForce=off  RzSenseUpperLimitTorqueForce=off
  Integrator : Integrator
  MATLAB Function : MATLAB Function  Commented=on  TreatAsAtomicUnit=on
  PS-Simulink Converter{,1..5} (6 alike) : nesl_utility/PS-Simulink Converter  PhysicalDomain=network_engine_domain  SubClassName=ps_output  LeftPortType=input  RightPortType=output  PseudoPeriodic=off  Frequencies=[]  VectorFormat=inherit  Unit=inherit  AffineConversion=off
  Rectangular Joint : sm_lib/Joints/Rectangular Joint  JointMode=Normal  CompositeWrenchDir=FollowerOnBase  CompositeWrenchFrame=BaseFrame  SenseConstraintForce=off  SenseConstraintTorque=off  SenseTotalForce=off  SenseTotalTorque=off  PxPositionTargetSpecify=off  PxPositionTargetPriority=High  PxPositionTargetValue=1  PxPositionTargetValueUnits=m  PxVelocityTargetSpecify=off  PxVelocityTargetPriority=High  PxVelocityTargetValue=0  PxVelocityTargetValueUnits=m/s  PxEquilibriumPosition=0  PxEquilibriumPositionUnits=m  PxSpringStiffness=0  PxSpringStiffnessUnits=N/m  PxDampingCoefficient=0  PxDampingCoefficientUnits=N/(m/s)  PxLowerLimitSpecify=off  PxLowerLimitBound=-1  PxLowerLimitBoundUnits=m  PxLowerLimitStiffness=1e6  PxLowerLimitStiffnessUnits=N/m  PxLowerLimitDamping=1e3  PxLowerLimitDampingUnits=N/(m/s)  PxLowerLimitTransitionRegionWidth=1e-4  PxLowerLimitTransitionRegionWidthUnits=m  PxUpperLimitSpecify=off  PxUpperLimitBound=1  PxUpperLimitBoundUnits=m  PxUpperLimitStiffness=1e6  PxUpperLimitStiffnessUnits=N/m  PxUpperLimitDamping=1e3  PxUpperLimitDampingUnits=N/(m/s)  PxUpperLimitTransitionRegionWidth=1e-4  PxUpperLimitTransitionRegionWidthUnits=m  PxTorqueActuationMode=NoTorque  PxMotionActuationMode=ComputedMotion  PxSensePosition=off  PxSenseVelocity=off  PxSenseAcceleration=off  PxSenseTorqueForce=off  PxSenseLowerLimitTorqueForce=off  PxSenseUpperLimitTorqueForce=off  PyPositionTargetSpecify=off  PyPositionTargetPriority=High  PyPositionTargetValue=0  PyPositionTargetValueUnits=m  PyVelocityTargetSpecify=off  PyVelocityTargetPriority=High  PyVelocityTargetValue=0  PyVelocityTargetValueUnits=m/s  PyEquilibriumPosition=0  PyEquilibriumPositionUnits=m  PySpringStiffness=0  PySpringStiffnessUnits=N/m  PyDampingCoefficient=0  PyDampingCoefficientUnits=N/(m/s)  PyLowerLimitSpecify=off  PyLowerLimitBound=-1  PyLowerLimitBoundUnits=m  PyLowerLimitStiffness=1e6  PyLowerLimitStiffnessUnits=N/m  PyLowerLimitDamping=1e3  PyLowerLimitDampingUnits=N/(m/s)  PyLowerLimitTransitionRegionWidth=1e-4  PyLowerLimitTransitionRegionWidthUnits=m  PyUpperLimitSpecify=off  PyUpperLimitBound=1  PyUpperLimitBoundUnits=m  PyUpperLimitStiffness=1e6  PyUpperLimitStiffnessUnits=N/m  PyUpperLimitDamping=1e3  PyUpperLimitDampingUnits=N/(m/s)  PyUpperLimitTransitionRegionWidth=1e-4  PyUpperLimitTransitionRegionWidthUnits=m  PyTorqueActuationMode=NoTorque  PyMotionActuationMode=ComputedMotion  PySensePosition=off  PySenseVelocity=off  PySenseAcceleration=off  PySenseTorqueForce=off  PySenseLowerLimitTorqueForce=off  PySenseUpperLimitTorqueForce=off
  Scope : Scope  NumInputPorts=2
  Scope1 : Scope  NumInputPorts=3
  Scope2 : Scope  NumInputPorts=2
  Scope3 : Scope  NumInputPorts=2
  Transform Sensor : sm_lib/Frames and Transforms/Transform Sensor  MeasurementFrame=World  RotationSequence=XYX  SenseAngle=off  SenseAxis=off  SenseQ=off  SenseR=off  SenseRotationSequence=off  SenseOmegaX=off  SenseOmegaY=off  SenseOmegaZ=off  SenseOmega=off  SenseQDot=off  SenseRDot=off  SenseRotationSequenceDot=off  SenseAlphaX=off  SenseAlphaY=off  SenseAlphaZ=off  SenseAlpha=off  SenseQDDot=off  SenseRDDot=off  SenseX=off  SenseY=off  SenseZ=off  SenseXYZ=off  SenseRad=off  SenseAzim=off  SenseDist=off  SenseInc=off  SenseXDot=on  SenseYDot=off  SenseZDot=off  SenseXYZDot=off  SenseRadDot=off  SenseAzimDot=off  SenseDistDot=off  SenseIncDot=off  SenseXDDot=off  SenseYDDot=off  SenseZDDot=off  SenseXYZDDot=off  SenseRadDDot=off  SenseAzimDDot=off  SenseDistDDot=off  SenseIncDDot=off
  body : sm_lib/Body Elements/Brick Solid  BrickDimensions=[0.25 0.14 0.4]  BrickDimensionsUnits=m  ExportEntireGeometry=on  InertiaType=CalculateFromGeometry  BasedOnType=Mass  Density=1000  DensityUnits=kg/m^3  Mass=14  MassUnits=kg  CenterOfMass=[0 0 0]  CenterOfMassUnits=m  MomentsOfInertia=[1 1 1]  MomentsOfInertiaUnits=kg*m^2  ProductsOfInertia=[0 0 0]  ProductsOfInertiaUnits=kg*m^2  GraphicType=FromGeometry  MarkerShape=Sphere  MarkerSize=10  GraphicVisPropType=SimpleVisualProperties  GraphicDiffuseColor=[0.4667 0.6745 0.1882]  GraphicOpacity=1  GraphicSpecularColor=[0.5 0.5 0.5 1.0]  GraphicAmbientColor=[0.15 0.15 0.15 1.0]  GraphicEmissiveColor=[0.0 0.0 0.0 1.0]  GraphicShininess=75  DoExposeReferenceFrame=on  SerializedFrames=<Frames/>
  ground : PMIOPort  Side=Left
  leg : PMIOPort  Port=2  Side=Right
  ψ : Outport
  Φ : Outport  Port=2
  d_Φ : Outport  Port=3
  θ_b : Outport  Port=4
  d_θ_b : Outport  Port=5
  d_s : Outport  Port=6
  s : Outport  Port=7
  wires:
  PS-Simulink Converter/1 -> Scope1/1, ψ/1
  PS-Simulink Converter1/1 -> Scope2/1, Scope1/2, Φ/1
  PS-Simulink Converter2/1 -> Scope2/2, d_Φ/1
  PS-Simulink Converter3/1 -> Scope/1, Scope1/3, θ_b/1
  PS-Simulink Converter4/1 -> Scope/2, d_θ_b/1
  PS-Simulink Converter5/1 -> Integrator/1, d_s/1, Scope3/1
  Integrator/1 -> s/1, Scope3/2
  connections:
  Rectangular Joint/RConn1 -- body/RConn1 -- Transform Sensor/RConn1 -- leg/RConn1
  ground/RConn1 -- Gimbal Joint/LConn1
  Gimbal Joint/RConn1 -- Transform Sensor/LConn1 -- Rectangular Joint/LConn1
  PS-Simulink Converter/LConn1 -- Gimbal Joint/RConn2
  PS-Simulink Converter1/LConn1 -- Gimbal Joint/RConn3
  PS-Simulink Converter2/LConn1 -- Gimbal Joint/RConn4
  PS-Simulink Converter3/LConn1 -- Gimbal Joint/RConn5
  PS-Simulink Converter4/LConn1 -- Gimbal Joint/RConn6
  PS-Simulink Converter5/LConn1 -- Transform Sensor/RConn2
